simulink model "oven_antiwindup"  (Simulink 7.4)
settings: Solver=ode45  StartTime=0.0  StopTime=1000  MaxStep=0.1  RelTol=1e-3
libraries: simulink x1
settings Model: Creator=psonna  LastModifiedBy=psonna

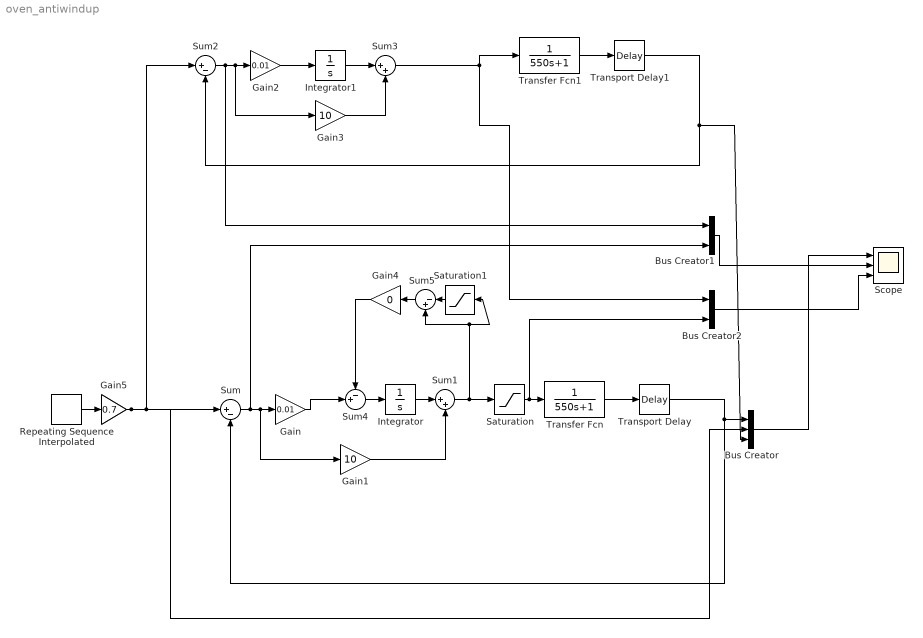
== system oven_antiwindup ==
  Bus Creator : BusCreator  Inputs=3
  Bus Creator1 : BusCreator  Inputs=2
  Bus Creator2 : BusCreator  Inputs=2
  Gain : Gain  Gain=0.01  ParameterDataType=fixdt(1, 16)  ParameterScaling=2^0  OutDataType=fixdt(1, 16)  OutScaling=2^0
  Gain1 : Gain  Gain=10  ParameterDataType=fixdt(1, 16)  ParameterScaling=2^0  OutDataType=fixdt(1, 16)  OutScaling=2^0
  Gain2 : Gain  Gain=0.01  ParameterDataType=fixdt(1, 16)  ParameterScaling=2^0  OutDataType=fixdt(1, 16)  OutScaling=2^0
  Gain3 : Gain  Gain=10  ParameterDataType=fixdt(1, 16)  ParameterScaling=2^0  OutDataType=fixdt(1, 16)  OutScaling=2^0
  Gain4 : Gain  Gain=0  ParameterDataType=fixdt(1, 16)  ParameterScaling=2^0  OutDataType=fixdt(1, 16)  OutScaling=2^0
  Gain5 : Gain  Gain=0.7  ParameterDataType=fixdt(1, 16)  ParameterScaling=2^0  OutDataType=fixdt(1, 16)  OutScaling=2^0
  Integrator : Integrator
  Integrator1 : Integrator
  Repeating Sequence Interpolated : simulink/Sources/Repeating Sequence Interpolated  SystemSampleTime=-1  OutValues=[0 0.6 0.8 0.8 0.6 0].'  TimeValues=[0 400 450 550 600 1000].'  LookUpMeth=Interpolation-Use End Values  tsamp=0.01  OutMin=[]  OutMax=[]  OutDataTypeStr=slDataTypeAndScale(('double'),('2^-10'))  OutputDataTypeScalingMode=Specify via dialog  OutDataType=double  OutScaling=2^-10
  Saturation : Saturate  UpperLimit=1  LowerLimit=0  OutDataType=fixdt(1, 16)  OutScaling=2^0
  Saturation1 : Saturate  UpperLimit=1  LowerLimit=0  OutDataType=fixdt(1, 16)  OutScaling=2^0
  Scope : Scope  NumInputPorts=3
      settings: YMin=0~-5~-5  YMax=0.5~5~5
  Sum : Sum  Inputs=|+-  OutDataType=fixdt(1, 16)  OutScaling=2^0
  Sum1 : Sum  Inputs=|++  OutDataType=fixdt(1, 16)  OutScaling=2^0
  Sum2 : Sum  Inputs=|+-  OutDataType=fixdt(1, 16)  OutScaling=2^0
  Sum3 : Sum  Inputs=|++  OutDataType=fixdt(1, 16)  OutScaling=2^0
  Sum4 : Sum  Inputs=-+|  OutDataType=fixdt(1, 16)  OutScaling=2^0
  Sum5 : Sum  Inputs=|-+  OutDataType=fixdt(1, 16)  OutScaling=2^0
  Transfer Fcn : TransferFcn  Denominator=[550 1]
  Transfer Fcn1 : TransferFcn  Denominator=[550 1]
  Transport Delay : TransportDelay  DelayTime=36
  Transport Delay1 : TransportDelay  DelayTime=36
  wires:
  Transfer Fcn/1 -> Transport Delay/1
  Repeating Sequence Interpolated/1 -> Gain5/1
  Bus Creator/1 -> Scope/1
  Transport Delay/1 -> Sum/2, Bus Creator/1
  Sum/1 -> Gain/1, Gain1/1, Bus Creator1/2
  Integrator/1 -> Sum1/1
  Sum1/1 -> Saturation/1, Sum5/2, Saturation1/1
  Gain1/1 -> Sum1/2
  Saturation/1 -> Transfer Fcn/1, Bus Creator2/2
  Transfer Fcn1/1 -> Transport Delay1/1
  Transport Delay1/1 -> Sum2/2, Bus Creator/3
  Sum2/1 -> Gain2/1, Gain3/1, Bus Creator1/1
  Gain2/1 -> Integrator1/1
  Integrator1/1 -> Sum3/1
  Sum3/1 -> Transfer Fcn1/1, Bus Creator2/1
  Gain3/1 -> Sum3/2
  Bus Creator1/1 -> Scope/2
  Sum4/1 -> Integrator/1
  Gain/1 -> Sum4/2
  Saturation1/1 -> Sum5/1
  Sum5/1 -> Gain4/1
  Gain4/1 -> Sum4/1
  Bus Creator2/1 -> Scope/3
  Gain5/1 -> Bus Creator/2, Sum/1, Sum2/1
